simulink model "BDot2"  (R2015b)
settings: Solver=ode45  StartTime=0.01  StopTime=tprop  RelTol=1e-3
values from neighbouring files (symbols this model uses):
  epsilon0 = q(2:4)    [SetUp.m]
  eta0 = q(1)    [SetUp.m]
  J = [(1/12)*m*h^2 0 0 ; 0 (1/12)*m*h^2 0; 0 0 .5*m*r^2]    [SetUp.m]
  Jinv = inv(J)    [SetUp.m]
  kd = -J*2*zeta*nf    [SetUp.m]
  mu = 398600    [COES2rvd.m]    (also in SetUp.m; test.m)
  rvect = invconvmat*rvectx    [COES2rvd.m]    (also in test.m = rvect')
  TcON = -1    [SetUp.m]
  Tcy = [0 kd(2,2)*(.5*mw*rw^2)*capOmega 0]    [SetUp.m]
  TcyON = 0    [SetUp.m]
  vvect = invconvmat*vvectx    [COES2rvd.m]    (also in test.m = vvect')
  wbn0 = DCM*w    [SetUp.m]
undefined symbols (not defined in the file or in its folder): IAU
libraries: aerolibtransform2 x3, aerolibgravity2 x1
settings Model: Creator=Trent  LastModifiedBy=morganyost
settings DataIOCC: SaveFormat=Array
settings HardwareCC: ProdBitPerPointer=32  ProdLargestAtomicFloat=None  ProdIntDivRoundTo=Undefined  ProdEndianess=Unspecified  ProdWordSize=32  ProdHWDeviceType=32-bit Generic
settings GRTTargetCC: GeneratePreprocessorConditionals=Disable all
settings ConfigComp: CovModelRefEnable=Off

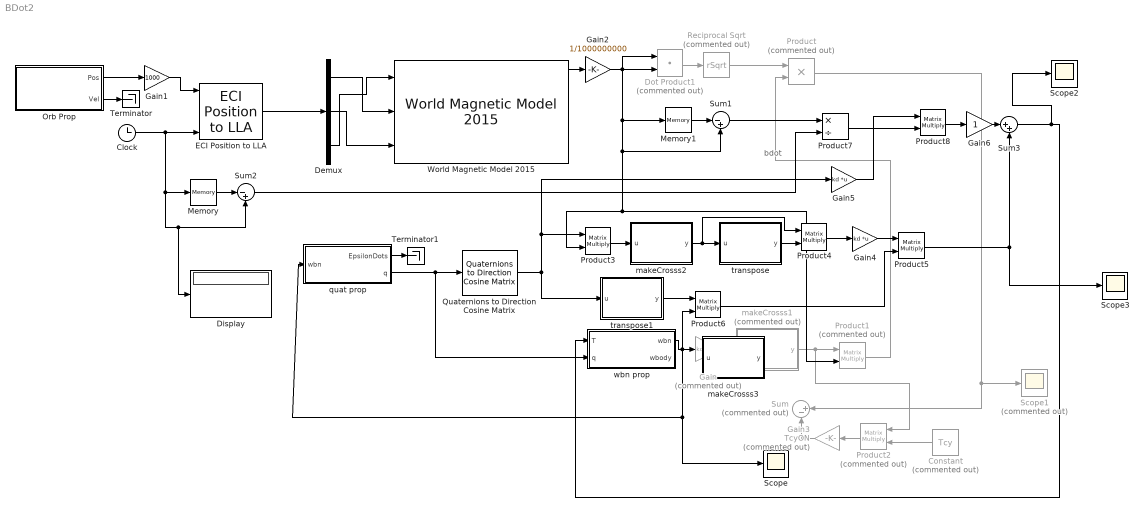
== system BDot2 ==
  note: bdot
  Clock : Clock
  Constant : Constant  Commented=on  Value=Tcy
  Demux : Demux  Outputs=3
  Display : Display
  Dot Product1 : DotProduct  Commented=on  InputSameDT=on  OutDataTypeStr=Inherit: Inherit via internal rule
  ECI Position to LLA : aerolibtransform2/ECI Position to LLA  red=IAU-2000/2006  year=2015  month=December  day=2  hour=0  min=0  sec=0  deltaT=Sec  errorflag=Error  extraparamflag=on  eunits=Metric (MKS)  earthmodel=WGS84  flat=1/298.257223563  eqradius=6378137
      settings: AttributesFormatString=%<red>
  Gain : Gain  Commented=on  Gain=kd  Multiplication=Matrix(K*u) (u vector)
  Gain1 : Gain  Gain=1000
  Gain2 : Gain  Gain=1/1000000000
  Gain3 : Gain  Commented=on  Gain=TcyON
  Gain4 : Gain  Gain=kd  Multiplication=Matrix(K*u)
  Gain5 : Gain  Gain=kd  Multiplication=Matrix(K*u)
  Gain6 : Gain
  Memory : Memory  X0=.0999999  InheritSampleTime=on
  Memory1 : Memory  X0=[2.1e-9;-5.8e-9;1e-9]  InheritSampleTime=on
  Orb Prop : Subsystem
  Product : Product  Commented=on
  Product1 : Product  Commented=on  Multiplication=Matrix(*)
  Product2 : Product  Commented=on  Multiplication=Matrix(*)
  Product{3..6,8} (5 alike) : Product  Multiplication=Matrix(*)
  Product7 : Product  Inputs=*/
  Quaternions to Direction Cosine Matrix : aerolibtransform2/Quaternions to  Direction Cosine Matrix
  Reciprocal Sqrt : Sqrt  Commented=on  Operator=rSqrt  SaturateOnIntegerOverflow=on
  Scope : Scope
  Scope1 : Scope  Commented=on
  Scope2 : Scope
  Scope3 : Scope
  Sum : Sum  Commented=on  Inputs=|+-
  Sum1 : Sum  Inputs=|-+
  Sum2 : Sum  Inputs=|-+
  Sum3 : Sum  Inputs=|++
  Terminator : Terminator
  Terminator1 : Terminator
  World Magnetic Model 2015 : aerolibgravity2/World Magnetic Model 2015  RequirementInfo="{}  %GIDa_c707c699_7679_46e8_b9d9_c8e087eee6a8"  units=Metric (MKS)  time_in=off  month=December  day=2  year=2015  action=Error  h_out=on  dec_out=on  inc_out=on  ti_out=on
  makeCrosss1 : MATLAB Function  Commented=on  TreatAsAtomicUnit=on
  makeCrosss2 : MATLAB Function  TreatAsAtomicUnit=on
  makeCrosss3 : MATLAB Function  TreatAsAtomicUnit=on
  quat prop : Subsystem
  transpose : MATLAB Function  TreatAsAtomicUnit=on
  transpose1 : MATLAB Function  TreatAsAtomicUnit=on
  wbn prop : Subsystem
  wires:
  ECI Position to LLA/1 -> Demux/1
  Clock/1 -> Memory/1, Display/1, Sum2/2, ECI Position to LLA/6
  Dot Product1/1 -> Reciprocal Sqrt/1
  Reciprocal Sqrt/1 -> Product/1
  wbn prop/1(wbn) -> Product6/2, quat prop/1(wbn), Scope/1, Gain/1
  Gain/1 -> makeCrosss1/1(u)
  makeCrosss1/1(y) -> Product2/1, Product1/1
  Product1/1 -> Product/2
  Product/1 -> Sum/1, Scope1/1
  Orb Prop/2(Vel) -> Terminator/1
  Demux/1 -> World Magnetic Model 2015/2
  Demux/2 -> World Magnetic Model 2015/3
  Demux/3 -> World Magnetic Model 2015/1
  Orb Prop/1(Pos) -> Gain1/1
  Gain1/1 -> ECI Position to LLA/1
  Constant/1 -> Product2/2
  Product2/1 -> Gain3/1
  Gain3/1 -> Sum/2
  quat prop/2(q) -> wbn prop/2(q), Quaternions to Direction Cosine Matrix/1
  quat prop/1(EpsilonDots) -> Terminator1/1
  Quaternions to Direction Cosine Matrix/1 -> transpose1/1(u), Product3/1, Gain5/1
  makeCrosss2/1(y) -> Product4/1, transpose/1(u)
  transpose/1(y) -> Product4/2
  Gain4/1 -> Product5/1
  Product3/1 -> makeCrosss2/1(u)
  transpose1/1(y) -> Product6/1
  Product6/1 -> Product5/2
  Memory/1 -> Sum2/1
  Sum2/1 -> Product7/2
  Sum1/1 -> Product7/1
  Product7/1 -> Product8/2
  Gain5/1 -> Product8/1
  Memory1/1 -> Sum1/1
  World Magnetic Model 2015/1 -> Gain2/1
  Sum3/1 -> Scope2/1, wbn prop/1(T)
  Product5/1 -> Sum3/2, Scope3/1
  Gain6/1 -> Sum3/1
  Product8/1 -> Gain6/1
  Product4/1 -> Gain4/1
  Gain2/1 -> Dot Product1/1, Dot Product1/2, Memory1/1, Sum1/2, Product3/2, Product1/2

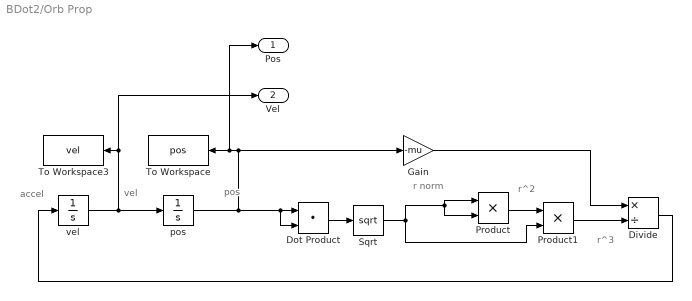
== system BDot2/Orb Prop ==
  note: r^3
  note: r^2
  note: r norm
  note: pos
  note: vel
  note: accel
  Divide : Product  Inputs=*/
  Dot Product : DotProduct  InputSameDT=on  OutDataTypeStr=Inherit: Inherit via internal rule
  Gain : Gain  Gain=-mu
  Product : Product
  Product1 : Product
  Sqrt : Sqrt  SaturateOnIntegerOverflow=on
  To Workspace : ToWorkspace  VariableName=pos  SaveFormat=Timeseries  SampleTime=-1
  To Workspace3 : ToWorkspace  VariableName=vel  SaveFormat=Timeseries  SampleTime=-1
  pos : Integrator  InitialCondition=rvect
  vel : Integrator  InitialCondition=vvect
  Pos : Outport
  Vel : Outport  Port=2
  wires:
  Sqrt/1 -> Product/2, Product/1, Product1/2
  Product/1 -> Product1/1
  Product1/1 -> Divide/2
  Gain/1 -> Divide/1
  Divide/1 -> vel/1
  Dot Product/1 -> Sqrt/1
  vel/1 -> Vel/1, To Workspace3/1, pos/1
  pos/1 -> Gain/1, Pos/1, To Workspace/1, Dot Product/2, Dot Product/1

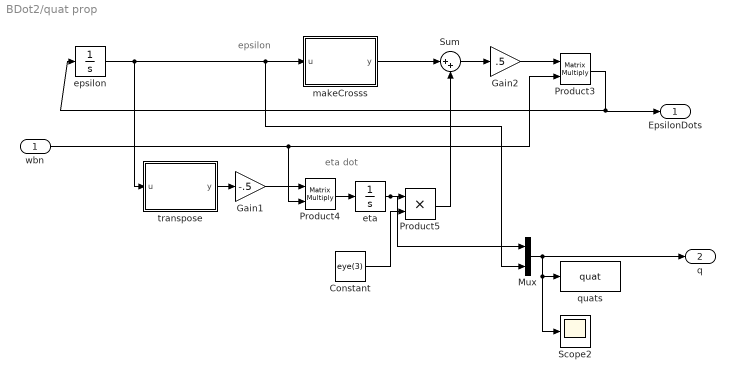
== system BDot2/quat prop ==
  note: eta dot
  note: epsilon
  wbn : Inport
  Constant : Constant  Value=eye(3)
  Gain1 : Gain  Gain=-.5
  Gain2 : Gain  Gain=.5
  Mux : Mux  Inputs=2
  Product3 : Product  Multiplication=Matrix(*)
  Product4 : Product  Multiplication=Matrix(*)
  Product5 : Product
  Scope2 : Scope
  Sum : Sum  Inputs=|++
  epsilon : Integrator  InitialCondition=epsilon0
  eta : Integrator  InitialCondition=eta0
  makeCrosss : MATLAB Function  TreatAsAtomicUnit=on
  quats : ToWorkspace  VariableName=quat  SaveFormat=Timeseries  SampleTime=-1
  transpose : MATLAB Function  TreatAsAtomicUnit=on
  EpsilonDots : Outport
  q : Outport  Port=2
  wires:
  epsilon/1 -> Mux/2, makeCrosss/1(u), transpose/1(u)
  makeCrosss/1(y) -> Sum/1
  eta/1 -> Mux/1, Product5/1
  Product5/1 -> Sum/2
  Sum/1 -> Gain2/1
  Gain2/1 -> Product3/1
  Product3/1 -> EpsilonDots/1, epsilon/1
  Product4/1 -> eta/1
  transpose/1(y) -> Gain1/1
  Constant/1 -> Product5/2
  Gain1/1 -> Product4/1
  Mux/1 -> q/1, quats/1, Scope2/1
  wbn/1 -> Product3/2, Product4/2

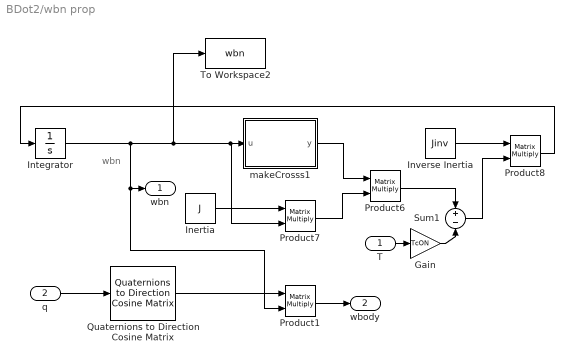
== system BDot2/wbn prop ==
  note: wbn
  T : Inport
  q : Inport  Port=2
  Gain : Gain  Gain=TcON
  Inertia : Constant  Value=J
  Integrator : Integrator  InitialCondition=wbn0
  Inverse Inertia : Constant  Value=Jinv
  Product{1,6..8} (4 alike) : Product  Multiplication=Matrix(*)
  Quaternions to Direction Cosine Matrix : aerolibtransform2/Quaternions to  Direction Cosine Matrix
  Sum1 : Sum  Inputs=+-
  To Workspace2 : ToWorkspace  VariableName=wbn  SaveFormat=Timeseries  SampleTime=-1
  makeCrosss1 : MATLAB Function  TreatAsAtomicUnit=on
  wbn : Outport
  wbody : Outport  Port=2
  wires:
  makeCrosss1/1(y) -> Product6/1
  Inertia/1 -> Product7/1
  Product7/1 -> Product6/2
  Inverse Inertia/1 -> Product8/1
  Product8/1 -> Integrator/1
  Product6/1 -> Sum1/1
  Sum1/1 -> Product8/2
  Integrator/1 -> Product1/2, wbn/1, Product7/2, makeCrosss1/1(u), To Workspace2/1
  T/1 -> Gain/1
  Gain/1 -> Sum1/2
  q/1 -> Quaternions to Direction Cosine Matrix/1
  Quaternions to Direction Cosine Matrix/1 -> Product1/1
  Product1/1 -> wbody/1

== matlab function BDot2/makeCrosss1 ==
  data: u input; y output
function y = fcn(u)
%#codegen
Ex = u(1);
Ey = u(2);
Ez = u(3);

y = [0 -Ez Ey; Ez 0 -Ex; -Ey Ex 0];

== matlab function BDot2/makeCrosss2 ==
  data: u input; y output
function y = fcn(u)
%#codegen
Ex = u(1);
Ey = u(2);
Ez = u(3);

y = [0 -Ez Ey; Ez 0 -Ex; -Ey Ex 0];

== matlab function BDot2/quat prop/makeCrosss ==
  data: u input; y output
function y = fcn(u)
%#codegen
Ex = u(1);
Ey = u(2);
Ez = u(3);

y = [0 -Ez Ey; Ez 0 -Ex; -Ey Ex 0];

== matlab function BDot2/wbn prop/makeCrosss1 ==
  data: u input; y output
function y = fcn(u)
%#codegen
Ex = u(1);
Ey = u(2);
Ez = u(3);

y = [0 -Ez Ey; Ez 0 -Ex; -Ey Ex 0];

== matlab function BDot2/transpose ==
  data: u input; y output
function y = fcn(u)
%#codegen

y = u';

== matlab function BDot2/quat prop/transpose ==
  data: u input; y output
function y = fcn(u)
%#codegen

y = u';

== matlab function BDot2/transpose1 ==
  data: u input; y output
function y = fcn(u)
%#codegen

y = u';

== matlab function BDot2/makeCrosss3 ==
  data: u input; y output
function y = fcn(u)
%#codegen
Ex = u(1);
Ey = u(2);
Ez = u(3);

y = [0 -Ez Ey; Ez 0 -Ex; -Ey Ex 0];
